simulink model "sl_ibvs"  (R2024b)
settings: Solver=ode45  StartTime=0.0  StopTime=10  RelTol=1e-3  EnableMultiTasking=on
InitFcn:
  | camera = CentralCamera('default')
undefined symbols (not defined in the file or in its folder): tformrz, trvec2tform
libraries: visualservolib x4, generallib x2, matrix_library x1
settings Model: Creator=pic  LastModifiedBy=pic
settings SolverCC: AlgebraicLoopSolver=TrustRegion
settings DataIOCC: SaveFormat=StructureWithTime  SignalLoggingSaveFormat=ModelDataLogs  DSMLogging=off
settings OptimizationCC: BlockReduction=off  BooleanDataType=off  ExpressionDepthLimit=2147483647  InitFltsAndDblsToZero=on  LifeSpan=inf
settings DebuggingCC: SaveWithParameterizedLinksMsg=none  UnderspecifiedInitializationDetection=Classic  MergeDetectMultiDrivingBlocksExec=none  SignalResolutionControl=TryResolveAllWithWarning  MultiTaskDSMMsg=warning  MultiTaskCondExecSysMsg=none  FcnCallInpInsideContextMsg=warning  UnconnectedInputMsg=warning  UnconnectedOutputMsg=warning  UnconnectedLineMsg=warning  AllowSymbolicDim=off  StateNameClashWarn=warning  SFUnexpectedBacktrackingDiag=warning  SFNoUnconditionalDefaultTransitionDiag=warning  SFExecutionAtInitializationDiag=none  ArithmeticOperatorsInVariantConditions=warning
settings HardwareCC: ProdBitPerPointer=32  ProdBitPerSizeT=32  ProdBitPerPtrDiffT=32  ProdLargestAtomicFloat=None  ProdIntDivRoundTo=Undefined  ProdEndianess=Unspecified  ProdWordSize=32  ProdHWDeviceType=32-bit Generic  TargetUnknown=on
settings ModelReferenceCC: EnableRefExpFcnMdlSchedulingChecks=on  PropagateSignalLabelsOutOfModel=off
settings SFSimCC: SimUseLocalCustomCode=off  CustomCodeUndefinedFunction=UseInterfaceOnly
settings RTWCC: RTWUseLocalCustomCode=off  GPUComputeCapability=3.5
settings CodeAppCC: StateflowObjectComments=on
settings GRTTargetCC: TargetLangStandard=C89/C90 (ANSI)  ModelReferenceCompliant=off  CompOptLevelCompliant=off  CombineOutputUpdateFcns=off  MatFileLogging=off  GRTInterface=on
settings ConfigComp: CovMetricSettings=dw  CovSaveCumulativeToWorkspaceVar=on  CovSaveSingleToWorkspaceVar=on  CovExternalEMLEnable=off

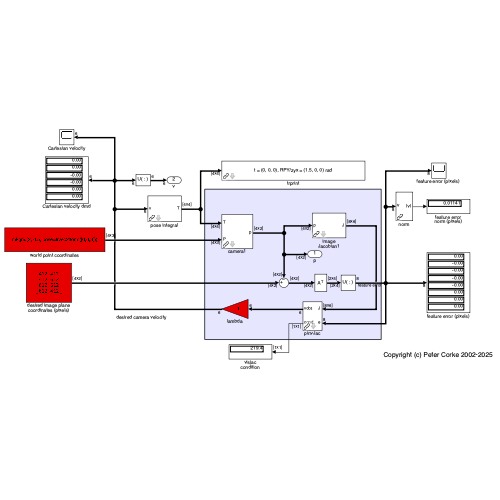
[thumbnail: Simulink's stored preview of the top-level diagram]
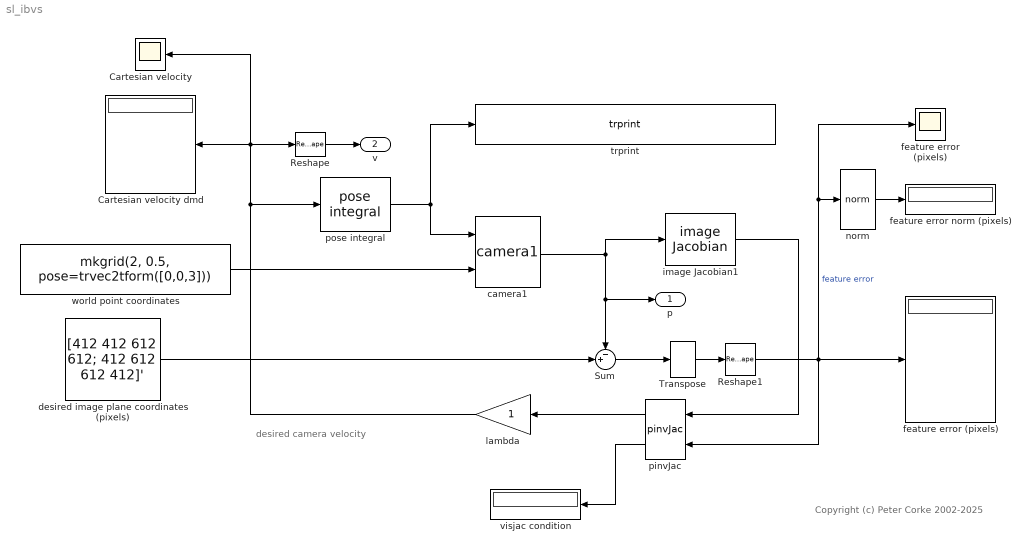
== system sl_ibvs ==
  note: Copyright (c) Peter Corke 2002-2025
  note: desired camera velocity
  Cartesian velocity : Scope
  Cartesian velocity dmd : Display
      settings: Format=bank
  Reshape : Reshape  OutputDimensions=6
  Reshape1 : Reshape  OutputDimensions=6
  Sum : Sum  Inputs=-+|  InputSameDT=on  SaturateOnIntegerOverflow=on  OutDataTypeStr=Inherit: Same as first input
  Transpose : matrix_library/Transpose
  camera1 : visualservolib/camera1  cam=camera
  desired image plane coordinates (pixels) : Constant  Value=[412 412 612 612; 412 612 612 412]'  VectorParams1D=off
  feature error norm (pixels) : Display
  feature error (pixels) : Display
      settings: Format=bank
  "feature error (pixels) " : Scope
  image Jacobian1 : visualservolib/image Jacobian  cam=camera  z=3
  lambda : Gain  SaturateOnIntegerOverflow=on  OutDataTypeStr=Inherit: Same as input  ParamDataTypeStr=Inherit: Same as input
  norm : generallib/norm  SystemSampleTime=-1  VariantActivationTime=update diagram  AllowFlexibleInterface=on  Latency=0  AutoFrameSizeCalculation=off
  pinvJac : visualservolib/pinvJac
  pose integral : visualservolib/pose integral  T0=trvec2tform([0,0,1])*tformrz(1.5)  dt=0.02
  trprint : generallib/trprint  options={}
  visjac condition : Display
  world point coordinates : Constant  Value=mkgrid(2, 0.5, pose=trvec2tform([0,0,3]))  VectorParams1D=off
  p : Outport
  v : Outport  Port=2
  wires:
  Sum/1 -> Transpose/1
  desired image plane coordinates (pixels)/1 -> Sum/2
  Reshape1/1 -> norm/1, "feature error (pixels) "/1, feature error (pixels)/1, pinvJac/2  "feature error"
  pinvJac/2 -> visjac condition/1
  pinvJac/1 -> lambda/1
  pose integral/1 -> camera1/1, trprint/1
  image Jacobian1/1 -> pinvJac/1
  lambda/1 -> pose integral/1, Cartesian velocity/1, Reshape/1, Cartesian velocity dmd/1
  Reshape/1 -> v/1
  camera1/1 -> image Jacobian1/1, Sum/1, p/1
  world point coordinates/1 -> camera1/2
  norm/1 -> feature error norm (pixels)/1
  Transpose/1 -> Reshape1/1
